simulink model "day2_local_control"  (R2022b)
settings: Solver=VariableStepAuto  StartTime=0.0  StopTime=10.0  RelTol=1e-3
undefined symbols (not defined in the file or in its folder): route1_waypoint_raw
libraries: CarMaker4SL x6
settings Model: Creator=USER  LastModifiedBy=USER

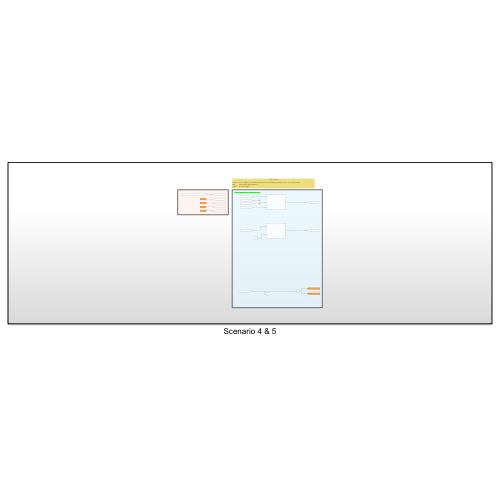
[thumbnail: Simulink's stored preview of the top-level diagram]
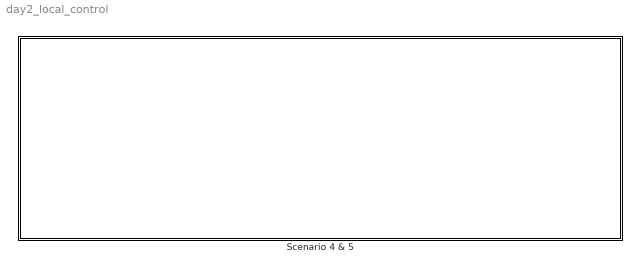
== system day2_local_control ==
  Scenario 4 & 5 : Subsystem

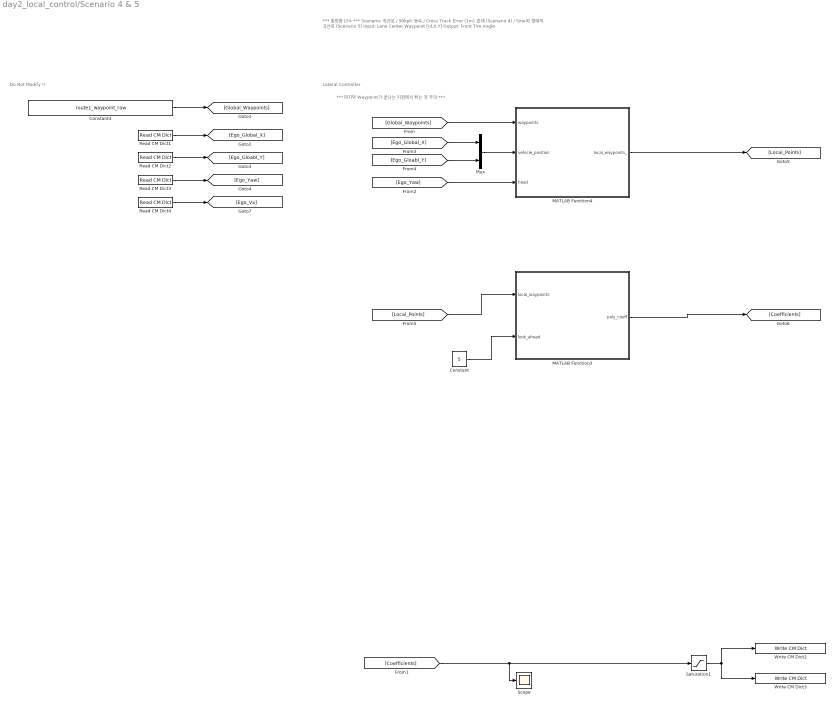
== system day2_local_control/Scenario 4 & 5 ==
  note: *** 마지막 Waypoint가 끝나는 지점에서 튀는 것 주의 ***
  note: Lateral Controller
  note: Do Not Modify !!
  note: *** 횡방향 LFA ***
      |
      | Scenario: 직선로 / 50kph 등속 / Cross Track Error (1m) 존재 (Scenario 4) / Sine파 형태의 곡선로 (Scenario 5)
      | Input: Lane Center Waypoint [id,X,Y]
      | Output: Front Tire Angle
  Constant : Constant  Value=5
  Constant4 : Constant  Value=route1_waypoint_raw
  MATLAB Function3 : MATLAB Function  TreatAsAtomicUnit=on
  "MATLAB Function4 " : MATLAB Function  TreatAsAtomicUnit=on
  Mux : Mux  Inputs=2
  Read CM Dict1 : CarMaker4SL/Read CM Dict  xname=Car.Fr1.tx  xsync=off  xstime=Inherited
  Read CM Dict2 : CarMaker4SL/Read CM Dict  xname=Car.Fr1.ty  xsync=off  xstime=Inherited
  Read CM Dict3 : CarMaker4SL/Read CM Dict  xname=Car.Fr1.rz  xsync=off  xstime=Inherited
  Read CM Dict4 : CarMaker4SL/Read CM Dict  xname=Car.v  xsync=off  xstime=Inherited
  Saturation1 : Saturate  UpperLimit=2  LowerLimit=-2
  Scope : Scope
  Write CM Dict2 : CarMaker4SL/Write CM Dict  xname=Car.CFL.rz_ext  xsync=off
  Write CM Dict3 : CarMaker4SL/Write CM Dict  xname=Car.CFR.rz_ext  xsync=off
  wires:
  Read CM Dict1/1 -> [Ego_Global_X]
  Read CM Dict2/1 -> [Ego_Gloabl_Y]
  Read CM Dict3/1 -> [Ego_Yaw]
  [Ego_Yaw] -> "MATLAB Function4 "/3(head)
  [Ego_Global_X] -> Mux/1
  [Ego_Gloabl_Y] -> Mux/2
  "MATLAB Function4 "/1(local_waypoints_) -> [Local_Points]
  [Global_Waypoints] -> "MATLAB Function4 "/1(waypoints)
  [Local_Points] -> MATLAB Function3/1(local_waypoints)
  MATLAB Function3/1(poly_coeff) -> [Coefficients]
  Saturation1/1 -> Write CM Dict2/1, Write CM Dict3/1
  Constant4/1 -> [Global_Waypoints]
  [Coefficients] -> Saturation1/1, Scope/1
  Mux/1 -> "MATLAB Function4 "/2(vehicle_position)
  Read CM Dict4/1 -> [Ego_Vx]
  Constant/1 -> MATLAB Function3/2(look_ahead)

== matlab function day2_local_control/Scenario 4 & 5/MATLAB Function3 ==
  settings: updateMethod=DISCRETE  sampleTime=0.05
  data: local_waypoints input; poly_coeff output; look_ahead input
function poly_coeff = fit_polynomial_to_waypoints(local_waypoints, look_ahead)
       
    filtered_matrix = local_waypoints(local_waypoints(:, 1) >= 0, :);

    % 3. 5번째 웨이포인트의 X, Y 좌표 가져오기
    X_5th = filtered_matrix(1, 1);  % 5번째 X 좌표
    Y_5th = filtered_matrix(1, 2);  % 5번째 Y 좌표
    
    % 4. 각도 계산 (X축을 기준으로 Y축 방향의 각도, 라디안 단위)
    if size(filtered_matrix, 1) > look_ahead
        temp = atan2(filtered_matrix(look_ahead, 2), filtered_matrix(look_ahead, 1));
    else
        temp = 0;
    end
    
    poly_coeff = atan2(Y_5th, 3) / 2 +  temp;  % atan2는 Y, X를 입력으로 받음
    scatter(filtered_matrix(:, 1), filtered_matrix(:, 2));
    xlim([-50, 50]);
    ylim([-50, 50]);
end

== matlab function day2_local_control/Scenario 4 & 5/MATLAB Function4  ==
  settings: updateMethod=DISCRETE  sampleTime=0.05
  data: waypoints input; local_waypoints_ output; vehicle_position input; head input
function local_waypoints_ = global_to_local_waypoints(waypoints, vehicle_position, head)
    num_waypoints = size(waypoints, 1);
    local_waypoints_ = zeros(num_waypoints, 2);

    % 헤딩 각에 대한 코사인 및 사인 계산
    cos_theta = cos(head);
    sin_theta = sin(head);

    for i = 1:num_waypoints
        % 글로벌 좌표에서 차량 위치를 빼서 상대적 위치 계산
        X_diff = waypoints(i, 1) - vehicle_position(1);
        Y_diff = waypoints(i, 2) - vehicle_position(2);
        
        % 2D 회전 변환을 통해 로컬 좌표로 변환
        local_waypoints_(i, 1) = X_diff * cos_theta + Y_diff * sin_theta;
        local_waypoints_(i, 2) = -X_diff * sin_theta + Y_diff * cos_theta;
    end
   
end
